simulink model "guidance"  (R2023a)
settings: Solver=ode4  StartTime=0.0  StopTime=10.0  FixedStep=dt  RelTol=1e-3
settings Model: Creator=hugobuurmeijer  LastModifiedBy=ndelurgio

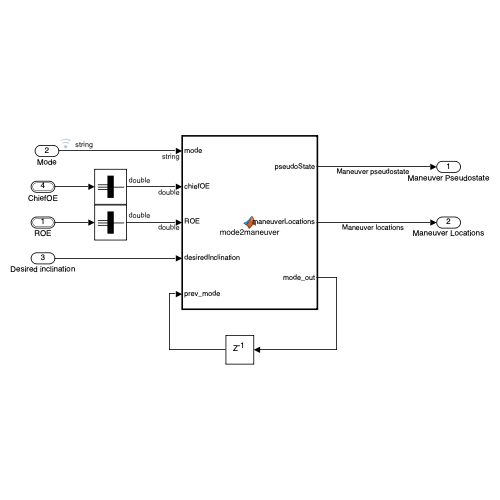
[thumbnail: Simulink's stored preview of the top-level diagram]
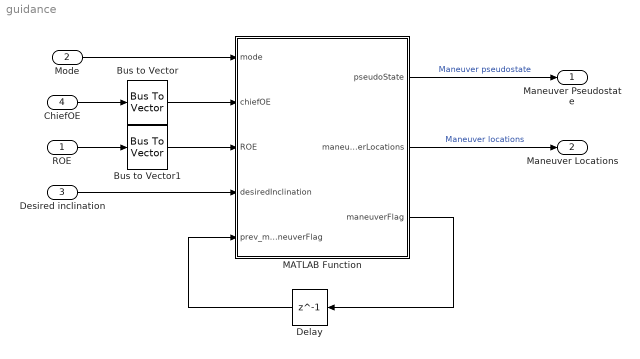
== system guidance ==
  ROE : Inport  OutDataTypeStr=Bus: eccentricSingularROE
  Mode : Inport  Port=2  OutDataTypeStr=string
  Desired inclination : Inport  Port=3  PortDimensions=2
  ChiefOE : Inport  Port=4  OutDataTypeStr=Bus: meanOrbitElements
  Bus to Vector : BusToVector
  Bus to Vector1 : BusToVector
  Delay : Delay  DelayLength=1  InitialCondition=0
  MATLAB Function : MATLAB Function  TreatAsAtomicUnit=on
  Maneuver Pseudostate : Outport
  Maneuver Locations : Outport  Port=2
  wires:
  ROE/1 -> Bus to Vector1/1
  Mode/1 -> MATLAB Function/1(mode)
  Desired inclination/1 -> MATLAB Function/4(desiredInclination)
  MATLAB Function/1(pseudoState) -> Maneuver Pseudostate/1  "Maneuver pseudostate"
  MATLAB Function/2(maneuverLocations) -> Maneuver Locations/1  "Maneuver locations"
  ChiefOE/1 -> Bus to Vector/1
  Bus to Vector/1 -> MATLAB Function/2(chiefOE)
  Bus to Vector1/1 -> MATLAB Function/3(ROE)
  MATLAB Function/3(maneuverFlag) -> Delay/1
  Delay/1 -> MATLAB Function/5(prev_maneuverFlag)

== matlab function guidance/MATLAB Function ==
  data: mode input; chiefOE input; pseudoState output; ROE input; desiredInclination input; maneuverLocations output [..69]; prev_maneuverFlag input; maneuverFlag output
function [pseudoState, maneuverLocations, maneuverFlag] = mode2maneuver(mode, chiefOE, ROE, desiredInclination, prev_maneuverFlag)

[pseudoState, maneuverLocations, maneuverFlag] = mode2maneuver(mode, chiefOE, ROE, desiredInclination, prev_maneuverFlag);

end
